simulink model "sampleModel2028"  (R2023a)
settings: Solver=VariableStepAuto  StartTime=0.0  StopTime=10.0  RelTol=1e-3
libraries: hdlsllib x2, simulink x1
settings Model: Creator=user1  LastModifiedBy=user1

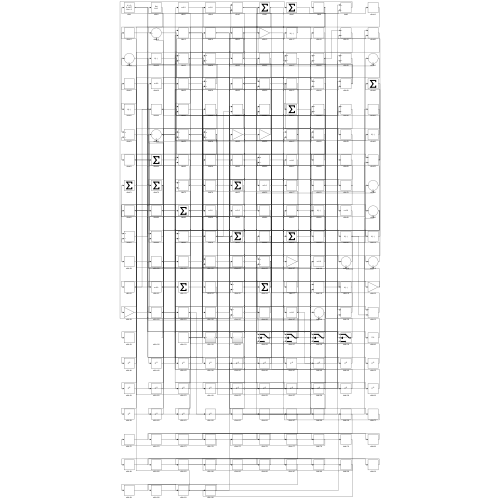
[thumbnail: Simulink's stored preview of the top-level diagram]
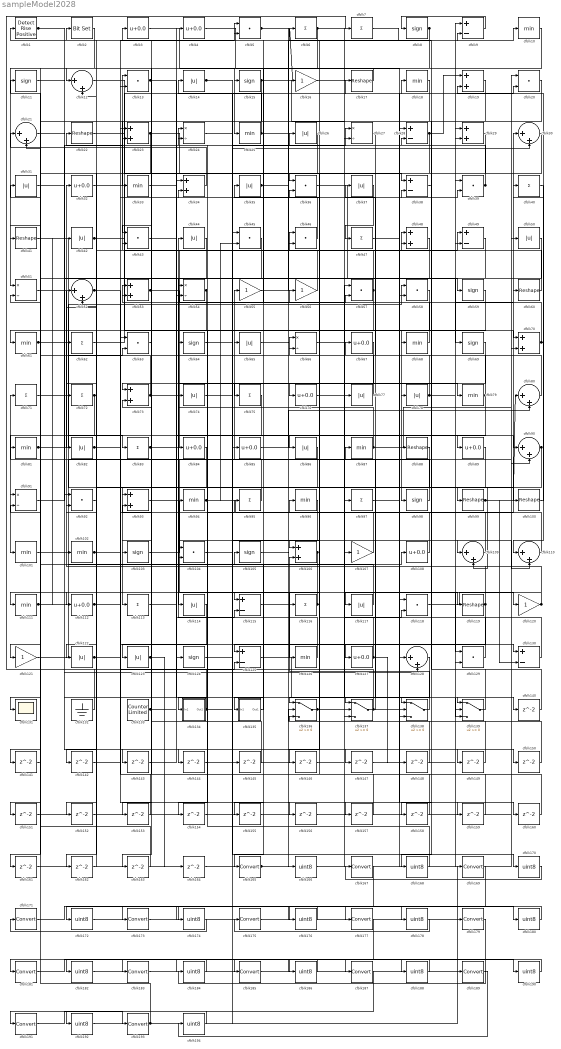
== system sampleModel2028 ==
  cfblk1 : hdlsllib/Logic and Bit Operations/Detect Rise Positive  vinit=0  OutDataTypeStr=boolean
  cfblk{10,18,25,33,61,68,79,81,87,94,96,101..102,111,126} (15 alike) : MinMax
  cfblk{17,22,41,60,88,99..100,119} (8 alike) : Reshape
  cfblk{8,11,15,59,64,69,98,103,105,124} (10 alike) : Signum
  cfblk{5,13,20,36,39,43,45..46,57..58,63,92,104,118,129} (15 alike) : DotProduct  OutDataTypeStr=Inherit: Inherit via internal rule
  cfblk{19,23,29,34,48,53,70,73,93,106} (10 alike) : Sum
  cfblk{16,55..56,107,120..121} (6 alike) : Gain
  cfblk{3..4,32,67,76,84..85,89,108,112,127} (11 alike) : Bias  Bias=0.0  SaturateOnIntegerOverflow=off
  cfblk{12,21,30,52,80,90,109..110,128} (9 alike) : Sum  Inputs=|++
  cfblk{6..7,40,47,62,71..72,75,83,95,97,113,116} (13 alike) : Sum  Inputs=+
  cfblk{14,26,31,35,37,42,44,50,65,74,77..78,82,86,114,117,122..123} (18 alike) : Abs  SaturateOnIntegerOverflow=off
  cfblk{9,28,38,49,115,125,130} (7 alike) : Sum  Inputs=+-
  cfblk131 : Scope
  cfblk132 : Ground
  cfblk133 : hdlsllib/Sources/Counter Limited  uplimit=7  tsamp=-1
  cfblk134 : Subsystem
      settings: LibrarySourceBlock=|
      | hdlsllib/Ports &
      | Subsystems/Subsystem
  cfblk135 : Subsystem
      settings: LibrarySourceBlock=|
      | hdlsllib/Ports &
      | Subsystems/Subsystem
  cfblk{136..139} (4 alike) : Switch  SaturateOnIntegerOverflow=off  InputSameDT=off
  cfblk{140..164} (25 alike) : Delay  SampleTime=1
  cfblk{165,167,169,171,173,175,177,179,181,183,185,187,189,191,193} (15 alike) : DataTypeConversion  SaturateOnIntegerOverflow=off  RndMeth=Floor
  cfblk{166,168,170,172,174,176,178,180,182,184,186,188,190,192,194} (15 alike) : DataTypeConversion  OutDataTypeStr=uint8  SaturateOnIntegerOverflow=off  RndMeth=Floor
  cfblk2 : simulink/Logic and Bit Operations/Bit Set  iBit=0
      settings: LibrarySourceBlock=|
      | hdlsllib/Logic and Bit
      | Operations/Bit Set
  cfblk{24,27,51,54,66,91} (6 alike) : Product  Inputs=*/  RndMeth=Zero  SaturateOnIntegerOverflow=on
  wires:
  cfblk119/1 -> cfblk125/1, cfblk102/1
  cfblk9/1 -> cfblk8/1
  cfblk121/1 -> cfblk108/1
  cfblk2/1 -> cfblk51/1
  cfblk7/1 -> cfblk10/1
  cfblk73/1 -> cfblk76/1, cfblk31/1
  cfblk95/1 -> cfblk71/1
  cfblk25/1 -> cfblk14/1, cfblk157/1
  cfblk135/1(Out1) -> cfblk105/1
  cfblk34/1 -> cfblk21/1
  cfblk94/1 -> cfblk30/1, cfblk110/2, cfblk45/2
  cfblk62/1 -> cfblk17/1
  cfblk139/1 -> cfblk67/1
  cfblk6/1 -> cfblk135/1(In1), cfblk139/2
  cfblk99/1 -> cfblk80/1, cfblk130/2
  cfblk102/1 -> cfblk95/1, cfblk144/1
  cfblk3/1 -> cfblk25/1
  cfblk30/1 -> cfblk106/1
  cfblk32/1 -> cfblk77/1
  cfblk41/1 -> cfblk99/1
  cfblk71/1 -> cfblk83/1
  cfblk124/1 -> cfblk49/1
  cfblk117/1 -> cfblk11/1
  cfblk125/1 -> cfblk139/1
  cfblk28/1 -> cfblk19/1, cfblk72/1
  cfblk56/1 -> cfblk13/1
  cfblk48/1 -> cfblk115/1
  cfblk59/1 -> cfblk98/1
  cfblk136/1 -> cfblk56/1, cfblk118/2
  cfblk68/1 -> cfblk53/1
  cfblk81/1 -> cfblk58/1, cfblk138/1, cfblk138/2
  cfblk118/1 -> cfblk120/1
  cfblk8/1 -> cfblk43/1, cfblk141/1
  cfblk66/1 -> cfblk119/1
  cfblk132/1 -> cfblk7/1
  cfblk29/1 -> cfblk86/1
  cfblk126/1 -> cfblk44/1
  cfblk100/1 -> cfblk19/2
  cfblk90/1 -> cfblk113/1, cfblk109/2, cfblk116/1
  cfblk12/1 -> cfblk36/1
  cfblk75/1 -> cfblk101/1
  cfblk77/1 -> cfblk55/1
  cfblk45/1 -> cfblk114/1
  cfblk67/1 -> cfblk73/1
  cfblk113/1 -> cfblk115/2
  cfblk17/1 -> cfblk12/1
  cfblk52/1 -> cfblk34/2, cfblk38/2, cfblk138/3
  cfblk16/1 -> cfblk59/1
  cfblk72/1 -> cfblk121/1, cfblk162/1
  cfblk138/1 -> cfblk106/2
  cfblk23/1 -> cfblk97/1, cfblk161/1
  cfblk36/1 -> cfblk69/1
  cfblk35/1 -> cfblk38/1, cfblk89/1
  cfblk61/1 -> cfblk63/2, cfblk23/2
  cfblk96/1 -> cfblk134/1(In1)
  cfblk38/1 -> cfblk78/1
  cfblk92/1 -> cfblk2/1
  cfblk79/1 -> cfblk91/1, cfblk37/1
  cfblk120/1 -> cfblk32/1, cfblk117/1
  cfblk51/1 -> cfblk82/1
  cfblk58/1 -> cfblk61/1
  cfblk130/1 -> cfblk66/1
  cfblk40/1 -> cfblk110/1
  cfblk60/1 -> cfblk22/1
  cfblk39/1 -> cfblk12/2, cfblk24/1
  cfblk85/1 -> cfblk80/2
  cfblk114/1 -> cfblk123/1
  cfblk83/1 -> cfblk29/1, cfblk90/1
  cfblk134/1(Out1) -> cfblk91/2, cfblk18/1
  cfblk54/1 -> cfblk84/1, cfblk131/1
  cfblk20/1 -> cfblk33/1
  cfblk70/1 -> cfblk35/1, cfblk40/1
  cfblk123/1 -> cfblk163/1, cfblk164/1
  cfblk137/1 -> cfblk52/2, cfblk87/1, cfblk140/1
  cfblk93/1 -> cfblk129/1
  cfblk87/1 -> cfblk20/1, cfblk24/2
  cfblk101/1 -> cfblk9/1
  cfblk103/1 -> cfblk65/1
  cfblk64/1 -> cfblk79/1
  cfblk42/1 -> cfblk46/2, cfblk152/1
  cfblk49/1 -> cfblk68/1
  cfblk106/1 -> cfblk154/1, cfblk155/1
  cfblk55/1 -> cfblk9/2
  cfblk27/1 -> cfblk137/1
  cfblk110/1 -> cfblk64/1
  cfblk53/1 -> cfblk57/2, cfblk139/3
  cfblk37/1 -> cfblk47/1
  cfblk116/1 -> cfblk111/1, cfblk96/1
  cfblk107/1 -> cfblk26/1
  cfblk115/1 -> cfblk126/1
  cfblk26/1 -> cfblk75/1
  cfblk91/1 -> cfblk62/1
  cfblk128/1 -> cfblk136/1
  cfblk22/1 -> cfblk85/1
  cfblk111/1 -> cfblk50/1, cfblk42/1
  cfblk10/1 -> cfblk15/1
  cfblk108/1 -> cfblk54/1
  cfblk21/1 -> cfblk92/1
  cfblk13/1 -> cfblk124/1, cfblk100/1
  cfblk4/1 -> cfblk128/1
  cfblk97/1 -> cfblk20/2
  cfblk88/1 -> cfblk165/1
  cfblk44/1 -> cfblk112/1
  cfblk78/1 -> cfblk3/1, cfblk60/1, cfblk158/1
  cfblk76/1 -> cfblk107/1
  cfblk112/1 -> cfblk5/1, cfblk150/1
  cfblk14/1 -> cfblk30/2, cfblk156/1
  cfblk80/1 -> cfblk48/1
  cfblk57/1 -> cfblk104/1, cfblk43/2
  cfblk122/1 -> cfblk125/2, cfblk159/1
  cfblk109/1 -> cfblk46/1
  cfblk46/1 -> cfblk5/2
  cfblk63/1 -> cfblk103/1
  cfblk133/1 -> cfblk4/1, cfblk48/2, cfblk39/2
  cfblk129/1 -> cfblk28/2
  cfblk98/1 -> cfblk73/2
  cfblk86/1 -> cfblk93/1
  cfblk104/1 -> cfblk27/1
  cfblk15/1 -> cfblk27/2, cfblk41/1
  cfblk33/1 -> cfblk70/1
  cfblk89/1 -> cfblk122/1
  cfblk5/1 -> cfblk16/1, cfblk127/1
  cfblk82/1 -> cfblk130/1, cfblk94/1
  cfblk43/1 -> cfblk54/2
  cfblk1/1 -> cfblk128/2, cfblk58/2
  cfblk127/1 -> cfblk6/1, cfblk148/1
  cfblk24/1 -> cfblk109/1
  cfblk140/1 -> cfblk1/1
  cfblk141/1 -> cfblk21/2
  cfblk84/1 -> cfblk142/1
  cfblk142/1 -> cfblk13/2
  cfblk31/1 -> cfblk143/1
  cfblk143/1 -> cfblk34/1
  cfblk144/1 -> cfblk57/1
  cfblk145/1 -> cfblk53/2
  cfblk69/1 -> cfblk146/1
  cfblk146/1 -> cfblk36/2
  cfblk105/1 -> cfblk147/1
  cfblk147/1 -> cfblk49/2
  cfblk148/1 -> cfblk136/3
  cfblk11/1 -> cfblk149/1
  cfblk149/1 -> cfblk28/1
  cfblk150/1 -> cfblk136/2
  cfblk50/1 -> cfblk151/1
  cfblk151/1 -> cfblk29/2
  cfblk152/1 -> cfblk52/1
  cfblk18/1 -> cfblk153/1
  cfblk153/1 -> cfblk63/1
  cfblk154/1 -> cfblk129/2
  cfblk155/1 -> cfblk137/2
  cfblk156/1 -> cfblk70/2
  cfblk157/1 -> cfblk23/1
  cfblk158/1 -> cfblk93/2
  cfblk159/1 -> cfblk104/2
  cfblk47/1 -> cfblk160/1
  cfblk160/1 -> cfblk66/2
  cfblk161/1 -> cfblk137/3
  cfblk162/1 -> cfblk92/2
  cfblk163/1 -> cfblk51/2
  cfblk164/1 -> cfblk45/1
  cfblk165/1 -> cfblk90/2, cfblk118/1, cfblk39/1
  cfblk65/1 -> cfblk166/1
  cfblk166/1 -> cfblk88/1
  cfblk19/1 -> cfblk168/1
  cfblk168/1 -> cfblk74/1
  cfblk74/1 -> cfblk170/1
  cfblk170/1 -> cfblk167/1
  cfblk167/1 -> cfblk172/1
  cfblk172/1 -> cfblk169/1
  cfblk169/1 -> cfblk174/1
  cfblk174/1 -> cfblk171/1
  cfblk171/1 -> cfblk176/1
  cfblk176/1 -> cfblk173/1
  cfblk173/1 -> cfblk178/1
  cfblk178/1 -> cfblk175/1
  cfblk175/1 -> cfblk180/1
  cfblk180/1 -> cfblk177/1
  cfblk177/1 -> cfblk182/1
  cfblk182/1 -> cfblk179/1
  cfblk179/1 -> cfblk184/1
  cfblk184/1 -> cfblk181/1
  cfblk181/1 -> cfblk186/1
  cfblk186/1 -> cfblk183/1
  cfblk183/1 -> cfblk188/1
  cfblk188/1 -> cfblk185/1
  cfblk185/1 -> cfblk190/1
  cfblk190/1 -> cfblk187/1
  cfblk191/1 -> cfblk193/1
  cfblk187/1 -> cfblk192/1
  cfblk192/1 -> cfblk189/1
  cfblk193/1 -> cfblk81/1, cfblk145/1
  cfblk189/1 -> cfblk194/1
  cfblk194/1 -> cfblk191/1

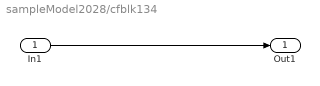
== system sampleModel2028/cfblk134 ==
  In1 : Inport
  Out1 : Outport
  wires:
  In1/1 -> Out1/1

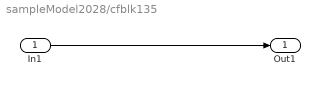
== system sampleModel2028/cfblk135 ==
  In1 : Inport
  Out1 : Outport
  wires:
  In1/1 -> Out1/1
